simulink model "RingModulator"  (R2019a)
settings: Solver=VariableStepAuto  StartTime=0.0  StopTime=15  RelTol=1e-3
libraries: dspvision x1, dspsrcs4 x1, dspobslib x1
settings Model: Creator=Ahmed  LastModifiedBy=Ahmed

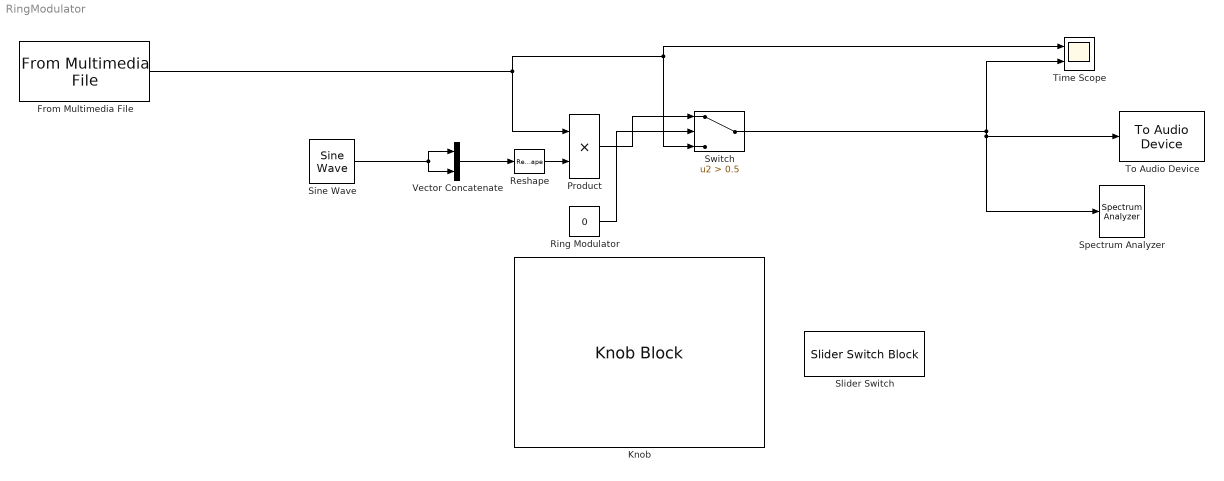
== system RingModulator ==
  From Multimedia File : dspvision/From Multimedia File  inputFilename=C:\Users\Ahmed\Nextcloud\L3\LU3EE105\Audio\Documents de TP et projet-20191118\Projet\atlas_air.wav  readRange=[1 Inf]  loop=on  numPlays=inf  outputStreams=Audio only  videoDataType=single  audioDataType=double  inheritSampleTime=on  userDefinedSampleTime=1/30  noAudioOutput=off  isIntensityVideo=off  fourcc=RGB  colorVideoFormat=Separate color signals  outputEOF=off  dataOrg=Column-major  audioFrameSize=1024  computeAudioFrameSize=off  outSamplingMode=Sample based
      settings: SourceProductName=DSP System Toolbox  SourceProductBaseCode=DS
  Knob : KnobBlock  ScaleMin=100  ScaleMax=2000
  Product : Product
  Reshape : Reshape  OutputDimensionality=Customize  OutputDimensions=[1024,2]
  Ring Modulator : Constant  Value=0
  Sine Wave : dspsrcs4/Sine Wave  Amplitude=1  Frequency=626.4678039550781  Phase=0  SampleMode=Discrete  OutComplex=Real  CompMethod=Trigonometric fcn  TableSize=Speed  SampleTime=1/48000  SamplesPerFrame=1024  ResetState=Restart at time zero  OutputFrames=off  dataType=double  wordLen=16  udDataType=sfix(16)  fracBitsMode=Best precision  numFracBits=15  OutDataTypeStr=double  LastOutDataTypeStr=double
  Slider Switch : SliderSwitchBlock
      settings: Values={{'Off', 'On'}, [0 1]}
  Spectrum Analyzer : SpectrumAnalyzer
  Switch : Switch  Criteria=u2 > Threshold  Threshold=0.5
  Time Scope : Scope  NumInputPorts=2
  To Audio Device : dspobslib/To Audio Device  deviceName=Default  inheritSampleRate=on  sampleRate=44100  deviceDatatype=Determine from input data type  autoBufferSize=on  bufferSize=4096  queueDuration=1.0  defaultOutputChannelMapping=on  outputChannelMapping=1:2  outputNumUnderrunSamples=off
      settings: SourceProductName=DSP System Toolbox  SourceProductBaseCode=DS
  Vector Concatenate : Concatenate
  wires:
  Switch/1 -> Time Scope/2, Spectrum Analyzer/1, To Audio Device/1
  Vector Concatenate/1 -> Reshape/1
  Reshape/1 -> Product/2
  From Multimedia File/1 -> Product/1, Switch/3, Time Scope/1
  Sine Wave/1 -> Vector Concatenate/2, Vector Concatenate/1
  Product/1 -> Switch/1
  Ring Modulator/1 -> Switch/2
